simulink model "Night_Detector"  (R2024a)
settings: Solver=FixedStepDiscrete  StartTime=0.0  StopTime=10.0  RelTol=1e-3  EnableMultiTasking=on
values from neighbouring files (symbols this model uses):
  Dem_EventStatusType : value not decoded    [dict.sldd]
libraries: autosarlibnvm x1, autosarlibdem x1
settings Model: DataDictionary=dict.sldd  Creator=Administrator  LastModifiedBy=Administrator
settings OptimizationCC: DefaultParameterBehavior=Inlined  EnhancedBackFolding=on  PassReuseOutputArgsAs=Individual arguments  ZeroExternalMemoryAtStartup=off  ZeroInternalMemoryAtStartup=off  OptimizeBlockOrder=speed  DifferentSizesBufferReuse=on  OptimizationCustomize=off  EfficientTunableParamExpr=on
settings DebuggingCC: ParameterTunabilityLossMsg=error
settings SFSimCC: MATLABDynamicMemAlloc=off
settings RTWCC: Description=AUTOSAR  SystemTargetFile=autosar.tlc  GenCodeOnly=on  TemplateMakefile=ert_default_tmf  DataTypeReplacement=CDataTypesFixedWidth
settings CodeAppCC: ForceParamTrailComments=on  IgnoreCustomStorageClasses=off  OperatorAnnotations=on  SimulinkDataObjDesc=on  SFDataObjDesc=on  InsertBlockDesc=on
settings STFCustomTargetCC: MultiwordLength=256  ParMdlRefBuildCompliant=on  CompOptLevelCompliant=on  IncludeMdlTerminateFcn=off  CombineOutputUpdateFcns=on  SuppressErrorStatus=on  ERTCustomFileBanners=on  SupportNonFinite=off  SupportComplex=off  SupportContinuousTime=off  SupportNonInlinedSFcns=off  RemoveResetFunc=on  MATLABClassNameForMDSCustomization=Simulink.SoftwareTarget.ERTCustomization  AutosarCompliant=on  GRTInterface=off  LookupTableObjectStructAxisOrder=2,1,3,4,...  LUTObjectStructOrderEvenSpacing=Size,Table,Breakpoints  SystemTargetFile=autosar.tlc
settings ERTTargetCC: TargetLangStandard=C99 (ISO)  ConcurrentExecutionCompliant=off  IncludeMdlTerminateFcn=off  SuppressErrorStatus=on  SupportNonFinite=off  SupportComplex=off  ModelStepFunctionPrototypeControlCompliant=off  CPPClassGenCompliant=off  AutosarCompliant=on  LookupTableObjectStructAxisOrder=2,1,3,4,...  LUTObjectStructOrderEvenSpacing=Size,Table,Breakpoints  InlinedParameterPlacement=NonHierarchical  ERTCustomFileTemplate=example_file_process.tlc  BooleanTrueId=TRUE  BooleanFalseId=FALSE

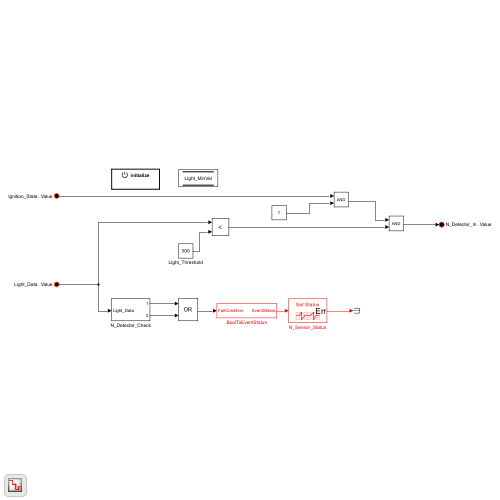
[thumbnail: Simulink's stored preview of the top-level diagram]
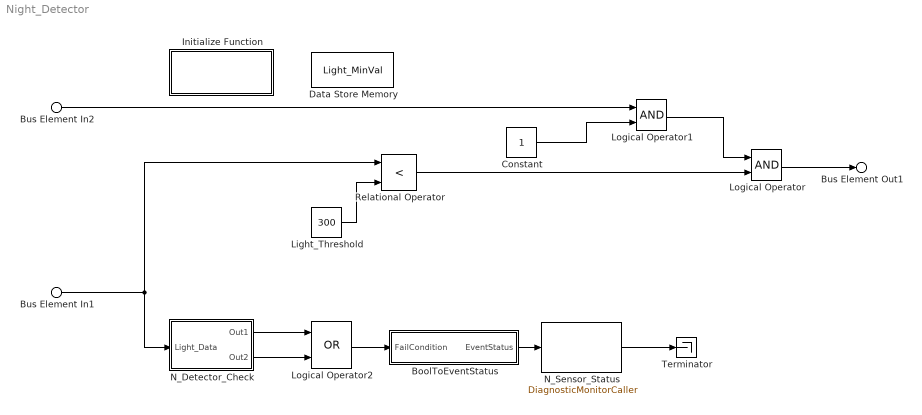
== system Night_Detector ==
  Bus Element In2 : Inport  Description=|  PortName=Ignition_State  Element=Value
      | Ignition State:
      | 0: OFF
      | 1: ON
  Bus Element In1 : Inport  Port=2  PortName=Light_Data  Element=Value
  BoolToEventStatus : Subsystem
  Constant : Constant  OutMin=0  OutMax=1  OutDataTypeStr=boolean
  Data Store Memory : DataStoreMemory  DataStoreName=Light_MinVal  WriteAfterWriteMsg=warning  ShowAdditionalParam=off
  Initialize Function : Subsystem  TreatAsAtomicUnit=on
  Light_Threshold : Constant  Value=300  OutMin=0  OutMax=50000  OutDataTypeStr=uint16
  Logical Operator : Logic  AllPortsSameDT=off  OutDataTypeStr=boolean
  Logical Operator1 : Logic  AllPortsSameDT=off  OutDataTypeStr=boolean
  Logical Operator2 : Logic  Operator=OR  AllPortsSameDT=off  OutDataTypeStr=boolean
  N_Detector_Check : Subsystem
  N_Sensor_Status : autosarlibdem/DiagnosticMonitorCaller  PortName=N_Detector  Operation=SetEventStatus  Datatype=Enum: Dem_EventStatusType  st=-1  ServiceImpl=autosar.bsw.DemDiagnosticMonitor  SyncToSchema=off
  Relational Operator : RelationalOperator  Operator=<  OutDataTypeStr=boolean  RndMeth=Simplest  InputSameDT=off
  Terminator : Terminator
  Bus Element Out1 : Outport  PortName=N_Detector_In  Element=Value
  wires:
  Light_Threshold/1 -> Relational Operator/2
  N_Sensor_Status/1 -> Terminator/1
  N_Detector_Check/1(Out1) -> Logical Operator2/1
  Bus Element In2/1 -> Logical Operator1/1
  Logical Operator/1 -> Bus Element Out1/1
  Relational Operator/1 -> Logical Operator/2
  Logical Operator2/1 -> BoolToEventStatus/1(FailCondition)
  Bus Element In1/1 -> N_Detector_Check/1(Light_Data), Relational Operator/1
  Logical Operator1/1 -> Logical Operator/1
  BoolToEventStatus/1(EventStatus) -> N_Sensor_Status/1
  Constant/1 -> Logical Operator1/2
  N_Detector_Check/2(Out2) -> Logical Operator2/2

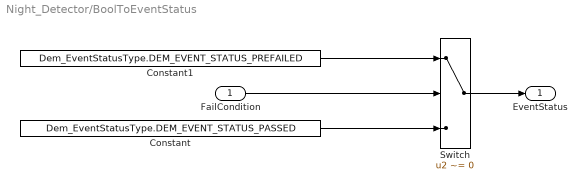
== system Night_Detector/BoolToEventStatus ==
  FailCondition : Inport
  Constant : Constant  Value=Dem_EventStatusType.DEM_EVENT_STATUS_PASSED
  Constant1 : Constant  Value=Dem_EventStatusType.DEM_EVENT_STATUS_PREFAILED
  Switch : Switch  Criteria=u2 ~= 0  SaturateOnIntegerOverflow=off  InputSameDT=off
  EventStatus : Outport  VectorParamsAs1DForOutWhenUnconnected=off
  wires:
  FailCondition/1 -> Switch/2
  Constant/1 -> Switch/3
  Constant1/1 -> Switch/1
  Switch/1 -> EventStatus/1

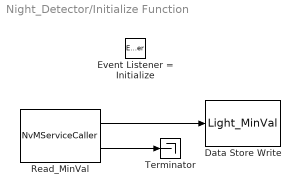
== system Night_Detector/Initialize Function ==
  Data Store Write : DataStoreWrite  DataStoreName=Light_MinVal  IndexOptions=Index vector (dialog)  Indices=1  OutputSizes=1
  "Event Listener = Initialize " : EventListener  DisableCoverage=on  EventName=reset
  Read_MinVal : autosarlibnvm/NvMServiceCaller  PortName=Light_MinVal  Operation=ReadBlock  ArgumentSpecification=uint16(0)  st=-1  ServiceImpl=autosar.bsw.NvMService  SyncToSchema=off
  Terminator : Terminator
  wires:
  Read_MinVal/1 -> Data Store Write/1
  Read_MinVal/2 -> Terminator/1

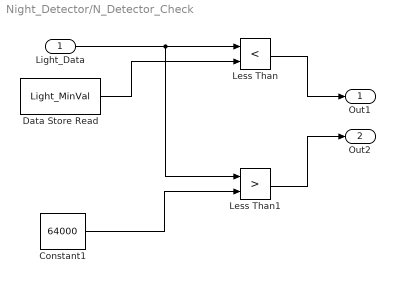
== system Night_Detector/N_Detector_Check ==
  Light_Data : Inport
  Constant1 : Constant  Value=64000
  Data Store Read : DataStoreRead  DataStoreName=Light_MinVal  IndexOptions=Index vector (dialog)  Indices=1  OutputSizes=1
  Less Than : RelationalOperator  Operator=<  OutDataTypeStr=boolean  RndMeth=Simplest  InputSameDT=off
  Less Than1 : RelationalOperator  Operator=>  OutDataTypeStr=boolean  RndMeth=Simplest  InputSameDT=off
  Out1 : Outport
  Out2 : Outport  Port=2
  wires:
  Data Store Read/1 -> Less Than/2
  Less Than1/1 -> Out2/1
  Light_Data/1 -> Less Than1/1, Less Than/1
  Constant1/1 -> Less Than1/2
  Less Than/1 -> Out1/1
